simulink model "HarmonicSeriesModel"  (R2021a)
settings: Solver=FixedStepAuto  StartTime=0.0  StopTime=10.0  FixedStep=.001  RelTol=1e-3
settings Model: Creator=ZZDDD  LastModifiedBy=ZZDDD
settings SolverCC: AlgebraicLoopSolver=TrustRegion
settings DataIOCC: LimitDataPoints=on  SaveOutput=off  SaveTime=off
settings OptimizationCC: BlockReduction=off  BooleanDataType=off  LifeSpan=inf
settings DebuggingCC: SaveWithParameterizedLinksMsg=none  UnderspecifiedInitializationDetection=Classic  MergeDetectMultiDrivingBlocksExec=none  SignalResolutionControl=TryResolveAllWithWarning  AllowSymbolicDim=off  SFUnexpectedBacktrackingDiag=warning  SFNoUnconditionalDefaultTransitionDiag=warning  SFExecutionAtInitializationDiag=none  SFMachineParentedDataDiag=warning  ArithmeticOperatorsInVariantConditions=warning
settings HardwareCC: TargetUnknown=on
settings SFSimCC: SimUseLocalCustomCode=off  CustomCodeUndefinedFunction=UseInterfaceOnly
settings RTWCC: RTWUseLocalCustomCode=off
settings CodeAppCC: StateflowObjectComments=on
settings GRTTargetCC: TargetLangStandard=C89/C90 (ANSI)

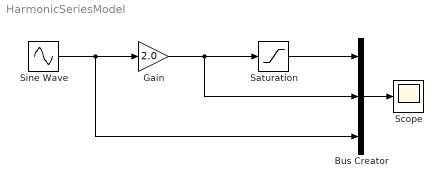
== system HarmonicSeriesModel ==
  Bus Creator : BusCreator  Inputs=3
  Gain : Gain  Gain=2.0
  Saturation : Saturate
  Scope : Scope
  Sine Wave : Sin  SampleTime=0
  wires:
  Gain/1 -> Bus Creator/2, Saturation/1
  Sine Wave/1 -> Bus Creator/3, Gain/1
  Bus Creator/1 -> Scope/1
  Saturation/1 -> Bus Creator/1
